simulink model "tests"  (R2019b)
settings: Solver=VariableStepAuto  StartTime=0.0  StopTime=15  RelTol=1e-3
settings Model: Creator=asmialek  LastModifiedBy=asmialek

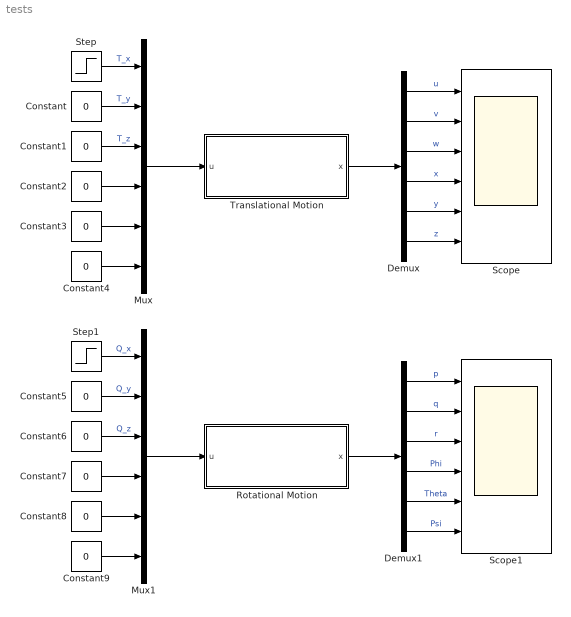
== system tests ==
  Constant{,1..9} (10 alike) : Constant  Value=0
  Demux : Demux  Outputs=6
  Demux1 : Demux  Outputs=6
  Mux : Mux  Inputs=6
  Mux1 : Mux  Inputs=6
  Rotational Motion : Subsystem
  Scope : Scope  NumInputPorts=6
  Scope1 : Scope  NumInputPorts=6
  Step : Step  Time=5  SampleTime=0
  Step1 : Step  Time=5  SampleTime=0
  Translational Motion : Subsystem
  wires:
  Step/1 -> Mux/1  "T_x"
  Constant/1 -> Mux/2  "T_y"
  Constant4/1 -> Mux/6
  Constant3/1 -> Mux/5
  Constant1/1 -> Mux/3  "T_z"
  Constant2/1 -> Mux/4
  Demux/1 -> Scope/1  "u"
  Demux/2 -> Scope/2  "v"
  Demux/3 -> Scope/3  "w"
  Demux/4 -> Scope/4  "x"
  Demux/5 -> Scope/5  "y"
  Demux/6 -> Scope/6  "z"
  Mux/1 -> Translational Motion/1(u)
  Translational Motion/1(x) -> Demux/1
  Step1/1 -> Mux1/1  "Q_x"
  Demux1/6 -> Scope1/6  "Psi"
  Constant8/1 -> Mux1/5
  Demux1/5 -> Scope1/5  "Theta"
  Demux1/3 -> Scope1/3  "r"
  Demux1/2 -> Scope1/2  "q"
  Constant7/1 -> Mux1/4
  Demux1/4 -> Scope1/4  "Phi"
  Demux1/1 -> Scope1/1  "p"
  Constant9/1 -> Mux1/6
  Constant5/1 -> Mux1/2  "Q_y"
  Rotational Motion/1(x) -> Demux1/1
  Constant6/1 -> Mux1/3  "Q_z"
  Mux1/1 -> Rotational Motion/1(u)

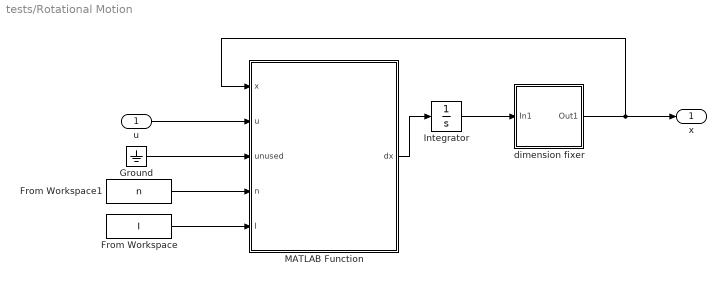
== system tests/Rotational Motion ==
  u : Inport
  From Workspace : FromWorkspace  VariableName=I  SampleTime=0
  From Workspace1 : FromWorkspace  VariableName=n  SampleTime=0
  Ground : Ground
  Integrator : Integrator
  MATLAB Function : MATLAB Function  TreatAsAtomicUnit=on
  dimension fixer : Subsystem
  x : Outport
  wires:
  Integrator/1 -> dimension fixer/1(In1)
  u/1 -> MATLAB Function/2(u)
  Ground/1 -> MATLAB Function/3(unused)
  MATLAB Function/1(dx) -> Integrator/1
  dimension fixer/1(Out1) -> x/1, MATLAB Function/1(x)
  From Workspace1/1 -> MATLAB Function/4(n)
  From Workspace/1 -> MATLAB Function/5(I)

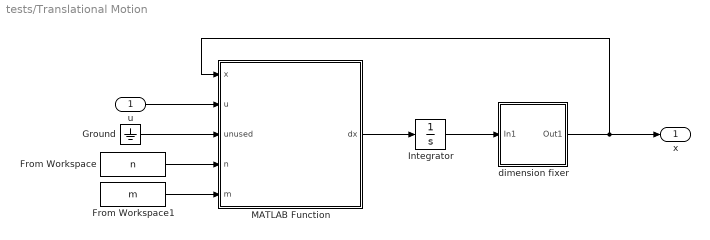
== system tests/Translational Motion ==
  u : Inport
  From Workspace : FromWorkspace  VariableName=n  SampleTime=0
  From Workspace1 : FromWorkspace  VariableName=m  SampleTime=0
  Ground : Ground
  Integrator : Integrator
  MATLAB Function : MATLAB Function  TreatAsAtomicUnit=on
  dimension fixer : Subsystem
  x : Outport
  wires:
  Integrator/1 -> dimension fixer/1(In1)
  u/1 -> MATLAB Function/2(u)
  Ground/1 -> MATLAB Function/3(unused)
  MATLAB Function/1(dx) -> Integrator/1
  dimension fixer/1(Out1) -> x/1, MATLAB Function/1(x)
  From Workspace/1 -> MATLAB Function/4(n)
  From Workspace1/1 -> MATLAB Function/5(m)

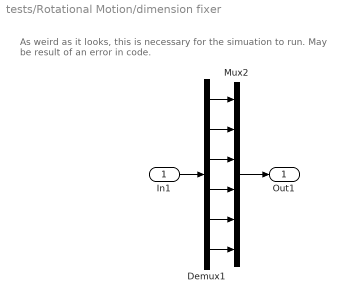
== system tests/Rotational Motion/dimension fixer ==
  note: As weird as it looks, this is necessary for the simuation to run.
      |
      | May be result of an error in code.
  In1 : Inport
  Demux1 : Demux  Outputs=6
  Mux2 : Mux  Inputs=6
  Out1 : Outport
  wires:
  Demux1/1 -> Mux2/1
  Demux1/5 -> Mux2/5
  Demux1/3 -> Mux2/3
  In1/1 -> Demux1/1
  Demux1/6 -> Mux2/6
  Demux1/2 -> Mux2/2
  Demux1/4 -> Mux2/4
  Mux2/1 -> Out1/1

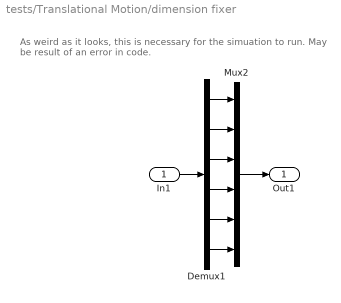
== system tests/Translational Motion/dimension fixer ==
  note: As weird as it looks, this is necessary for the simuation to run.
      |
      | May be result of an error in code.
  In1 : Inport
  Demux1 : Demux  Outputs=6
  Mux2 : Mux  Inputs=6
  Out1 : Outport
  wires:
  Demux1/1 -> Mux2/1
  Demux1/5 -> Mux2/5
  Demux1/3 -> Mux2/3
  In1/1 -> Demux1/1
  Demux1/6 -> Mux2/6
  Demux1/2 -> Mux2/2
  Demux1/4 -> Mux2/4
  Mux2/1 -> Out1/1

== matlab function tests/Rotational Motion/MATLAB Function ==
  data: x input; u input; dx output; unused input; n input; I input
function dx = translational_motion(x, u, ~, n, I)

        p = x(1);
        q = x(2);
        r = x(3);
      phi = x(4);
    theta = x(5);
      psi = x(6);

    G = [ 1  0          -sin(theta)           ;
          0  cos(theta)  cos(theta)*sin(phi)  ;
          0 -sin(theta)  cos(theta)*cos(phi) ];

    F = [ sin(psi)*cos(theta)                               ;
          sin(psi)*sin(theta)*sin(phi) + cos(psi)*cos(phi)  ;
          sin(psi)*sin(theta)*cos(phi) - cos(psi)*sin(phi) ];

    euler_derivatives = (G^-1)*([p q r]' + F.*n);

    p_dot = u(1) + (I(2) - I(3))*q*r;
    q_dot = u(2) + (I(3) - I(1))*r*p;
    r_dot = u(3) + (I(1) - I(2))*p*q;
    
    dx = [p_dot; q_dot; r_dot; euler_derivatives];
end

== matlab function tests/Translational Motion/MATLAB Function ==
  data: x input; u input; dx output; unused input; n input; m input
function dx = translational_motion(x, u, ~, n, m)

    A = [  0   0   n  -n^2 0   0     ;
           0   0   0   0  -n^2 0     ;
          -n   0   0   0   0   2*n^2 ;
           1   0   0   0   0   n     ;
           0   1   0   0   0   0     ;
           0   0   1  -n   0   0    ];

    B = [  1/m 0   0   0   0   0     ;
           0   1/m 0   0   0   0     ;
           0   0   1/m 0   0   0     ;
           0   0   0   0   0   0     ;
           0   0   0   0   0   0     ;
           0   0   0   0   0   0    ];        

    dx = A*x + B*u;
end
